simulink model "MotionLab_DigitalTwin"  (R2024b)
settings: Solver=ode3  StartTime=0.0  StopTime=inf  FixedStep=Ts  RelTol=1e-3  AbsTol=1e-3
model workspace: external: MATLAB File .\Parameters.m (data not in the file)
values from neighbouring files (symbols this model uses):
  L2 = 830e-3    (= 0.83)    [Robot_parameters.m]
  L3 = 1160e-3    (= 1.16)    [Robot_parameters.m]
  L4 = 250e-3    (= 0.25)    [Robot_parameters.m]
undefined symbols (not defined in the file or in its folder): smiData, smiDataBig, smiDataBigTop, smiDataRobot, Var, X, Y, Z
libraries: sm_lib x490, nesl_utility x87, slrealtimeutilitieslib x1, slrealtimeiplib x1, aerolibanimutils x1
(part 4 of 15)

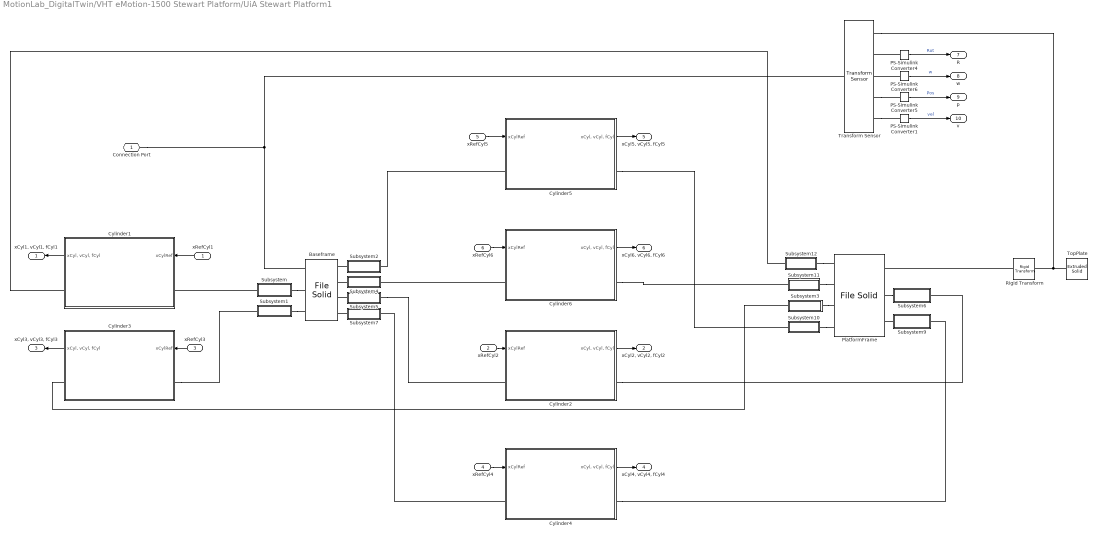
== system MotionLab_DigitalTwin/VHT eMotion-1500 Stewart Platform/UiA Stewart Platform1 ==
  xRefCyl1 : Inport
  xRefCyl2 : Inport  Port=2
  xRefCyl3 : Inport  Port=3
  xRefCyl4 : Inport  Port=4
  xRefCyl5 : Inport  Port=5
  xRefCyl6 : Inport  Port=6
  Baseframe : sm_lib/Body Elements/File Solid  ExtGeomFileName=.\CAD_Lille\1400_Derived Baseframe_crdincl.stp_Default_sldprt.STEP  UnitType=FromFile  ExtGeomFileUnits=m  StepReaderType=HEX  ExportConvexHullGeometry=off  InertiaType=Custom  BasedOnType=DensityFromFile  Density=1000  DensityUnits=kg/m^3  Mass=smiData.Solid(2).mass  MassUnits=kg  CenterOfMass=smiData.Solid(2).CoM  CenterOfMassUnits=mm  MomentsOfInertia=smiData.Solid(2).MoI  MomentsOfInertiaUnits=kg*mm^2  ProductsOfInertia=smiData.Solid(2).PoI  ProductsOfInertiaUnits=kg*mm^2  GraphicType=FromGeometry  MarkerShape=Sphere  MarkerSize=10  GraphicVisPropType=SimpleVisualProperties  GraphicDiffuseColor=[0.2 0.2 0.2]  GraphicOpacity=smiData.Solid(2).opacity  GraphicSpecularColor=[0.5 0.5 0.5 1.0]  GraphicAmbientColor=[0.15 0.15 0.15 1.0]  GraphicEmissiveColor=[0.0 0.0 0.0 1.0]  GraphicShininess=75  DoExposeReferenceFrame=on  SerializedFrames=<Frames><Frame><Id>Frame1</Id><Value><Name>F1</Name><Origin><Source>GeometricFeature</Source><FeatureName>planar surface 569</FeatureName></Origin><PrimaryAxis><DefinedDirection>+Z</DefinedDirection><Source>GeometricFeature</Source><SourceDirection>+Z</SourceDirection><FeatureName>planar surface 569</FeatureName></PrimaryAxis><SecondaryAxis><DefinedDirection>+X</DefinedDirection><Source>ReferenceFrame</Source><SourceDirection>+X</SourceDirection><FeatureName></FeatureName></SecondaryAxis></Value></Frame><Frame><Id>Frame2</Id><Value><Name>F2</Name><Origin><Source>GeometricFeature</Source><FeatureName>planar surface 568</FeatureName></Origin><PrimaryAxis><DefinedDirection>+Z</DefinedDirection><Source>GeometricFeature</Source><SourceDirection>+Z</SourceDirection><FeatureName>planar surface 568</FeatureName></PrimaryAxis><SecondaryAxis><DefinedDirection>+X</DefinedDirection><Source>ReferenceFrame</Source><SourceDirection>+X</SourceDirection><FeatureName></FeatureName></SecondaryAxis></Value></Frame><Frame><Id>Frame3</Id><Value><Name>F3</Name><Origin><Source>GeometricFeature</Source><FeatureName>planar surface 1053</FeatureName></Origin><PrimaryAxis><DefinedDirection>+Z</DefinedDirection><Source>GeometricFeature</Source><SourceDirection>+Z</SourceDirection><FeatureName>planar surface 1053</FeatureName></PrimaryAxis><SecondaryAxis><DefinedDirection>+X</DefinedDirection><Source>ReferenceFrame</Source><SourceDirection>+X</SourceDirection><FeatureName></FeatureName></SecondaryAxis></Value></Frame><Frame><Id>Frame4</Id><Value><Name>F4</Name><Origin><Source>GeometricFeature</Source><FeatureName>planar surface 1052</FeatureName></Origin><PrimaryAxis><DefinedDirection>+Z</DefinedDirection><Source>GeometricFeature</Source><SourceDirection>+Z</SourceDirection><FeatureName>planar surface 1052</FeatureName></PrimaryAxis><SecondaryAxis><DefinedDirection>+X</DefinedDirection><Source>ReferenceFrame</Source><SourceDirection>+X</SourceDirection><FeatureName></FeatureName></SecondaryAxis></Value></Frame><Frame><Id>Frame5</Id><Value><Name>F5</Name><Origin><Source>GeometricFeature</Source><FeatureName>planar surface 907</FeatureName></Origin><PrimaryAxis><DefinedDirection>+Z</DefinedDirection><Source>GeometricFeature</Source><SourceDirection>+Z</SourceDirection><FeatureName>planar surface 907</FeatureName></PrimaryAxis><SecondaryAxis><DefinedDirection>+X</DefinedDirection><Source>ReferenceFrame</Source><SourceDirection>+X</SourceDirection><FeatureName></FeatureName></SecondaryAxis></Value></Frame><Frame><Id>Frame6</Id><Value><Name>F6</Name><Origin><Source>GeometricFeature</Source><FeatureName>planar surface 906</FeatureName></Origin><PrimaryAxis><DefinedDirection>+Z</DefinedDirection><Source>GeometricFeature</Source><SourceDirection>+Z</SourceDirection><FeatureName>planar surface 906</FeatureName></PrimaryAxis><SecondaryAxis><DefinedDirection>+X</DefinedDirection><Source>ReferenceFrame</Source><SourceDirection>+X</SourceDirection><FeatureName></FeatureName></SecondaryAxis></Value></Frame></Frames>
  Cylinder1 : Subsystem
  Cylinder2 : Subsystem
  Cylinder3 : Subsystem
  Cylinder4 : Subsystem
  Cylinder5 : Subsystem
  Cylinder6 : Subsystem
  PS-Simulink Converter{1,4..6} (4 alike) : nesl_utility/PS-Simulink Converter  PhysicalDomain=network_engine_domain  SubClassName=ps_output  LeftPortType=input  RightPortType=output  PseudoPeriodic=off  Frequencies=[]  VectorFormat=inherit  Unit=inherit  AffineConversion=off
  PlatformFrame : sm_lib/Body Elements/File Solid  ExtGeomFileName=.\CAD_Lille\1100_Derived Platfrom_crdincl.stp_Default_sldprt.STEP  UnitType=FromFile  ExtGeomFileUnits=m  StepReaderType=HEX  ExportConvexHullGeometry=off  InertiaType=Custom  BasedOnType=DensityFromFile  Density=1000  DensityUnits=kg/m^3  Mass=smiData.Solid(4).mass  MassUnits=kg  CenterOfMass=smiData.Solid(4).CoM  CenterOfMassUnits=mm  MomentsOfInertia=smiData.Solid(4).MoI  MomentsOfInertiaUnits=kg*mm^2  ProductsOfInertia=smiData.Solid(4).PoI  ProductsOfInertiaUnits=kg*mm^2  GraphicType=FromGeometry  MarkerShape=Sphere  MarkerSize=10  GraphicVisPropType=SimpleVisualProperties  GraphicDiffuseColor=[0.2 0.2 0.2]  GraphicOpacity=1  GraphicSpecularColor=[0.5 0.5 0.5 1.0]  GraphicAmbientColor=[0.15 0.15 0.15 1.0]  GraphicEmissiveColor=[0.0 0.0 0.0 1.0]  GraphicShininess=75  DoExposeReferenceFrame=on  SerializedFrames=<Frames><Frame><Id>Frame1</Id><Value><Name>F1</Name><Origin><Source>GeometricFeature</Source><FeatureName>planar surface 875</FeatureName></Origin><PrimaryAxis><DefinedDirection>+Z</DefinedDirection><Source>GeometricFeature</Source><SourceDirection>+Z</SourceDirection><FeatureName>planar surface 875</FeatureName></PrimaryAxis><SecondaryAxis><DefinedDirection>+X</DefinedDirection><Source>ReferenceFrame</Source><SourceDirection>+X</SourceDirection><FeatureName></FeatureName></SecondaryAxis></Value></Frame><Frame><Id>Frame2</Id><Value><Name>F2</Name><Origin><Source>GeometricFeature</Source><FeatureName>planar surface 858</FeatureName></Origin><PrimaryAxis><DefinedDirection>+Z</DefinedDirection><Source>GeometricFeature</Source><SourceDirection>+Z</SourceDirection><FeatureName>planar surface 858</FeatureName></PrimaryAxis><SecondaryAxis><DefinedDirection>+X</DefinedDirection><Source>ReferenceFrame</Source><SourceDirection>+X</SourceDirection><FeatureName></FeatureName></SecondaryAxis></Value></Frame><Frame><Id>Frame3</Id><Value><Name>F3</Name><Origin><Source>GeometricFeature</Source><FeatureName>planar surface 428</FeatureName></Origin><PrimaryAxis><DefinedDirection>+Z</DefinedDirection><Source>GeometricFeature</Source><SourceDirection>+Z</SourceDirection><FeatureName>planar surface 428</FeatureName></PrimaryAxis><SecondaryAxis><DefinedDirection>+X</DefinedDirection><Source>ReferenceFrame</Source><SourceDirection>+X</SourceDirection><FeatureName></FeatureName></SecondaryAxis></Value></Frame><Frame><Id>Frame4</Id><Value><Name>F4</Name><Origin><Source>GeometricFeature</Source><FeatureName>planar surface 274</FeatureName></Origin><PrimaryAxis><DefinedDirection>+Z</DefinedDirection><Source>GeometricFeature</Source><SourceDirection>+Z</SourceDirection><FeatureName>planar surface 274</FeatureName></PrimaryAxis><SecondaryAxis><DefinedDirection>+X</DefinedDirection><Source>ReferenceFrame</Source><SourceDirection>+X</SourceDirection><FeatureName></FeatureName></SecondaryAxis></Value></Frame><Frame><Id>Frame5</Id><Value><Name>F5</Name><Origin><Source>GeometricFeature</Source><FeatureName>planar surface 892</FeatureName></Origin><PrimaryAxis><DefinedDirection>+Z</DefinedDirection><Source>GeometricFeature</Source><SourceDirection>+Z</SourceDirection><FeatureName>planar surface 892</FeatureName></PrimaryAxis><SecondaryAxis><DefinedDirection>+X</DefinedDirection><Source>ReferenceFrame</Source><SourceDirection>+X</SourceDirection><FeatureName></FeatureName></SecondaryAxis></Value></Frame><Frame><Id>Frame6</Id><Value><Name>F6</Name><Origin><Source>GeometricFeature</Source><FeatureName>planar surface 909</FeatureName></Origin><PrimaryAxis><DefinedDirection>+Z</DefinedDirection><Source>GeometricFeature</Source><SourceDirection>+Z</SourceDirection><FeatureName>planar surface 909</FeatureName></PrimaryAxis><SecondaryAxis><DefinedDirection>+X</DefinedDirection><Source>ReferenceFrame</Source><SourceDirection>+X</SourceDirection><FeatureName></FeatureName></SecondaryAxis></Value></Frame></Frames>
  Rigid Transform : sm_lib/Frames and Transforms/Rigid Transform  RotationMethod=None  FollAlignAxisA=+X  BaseAlignAxisA=+Y  FollAlignAxisB=+Y  BaseAlignAxisB=+Z  RotationStandardAxis=+Z  RotationAngle=0.0  RotationAngleUnits=deg  RotationArbitraryAxis=[0 0 1]  RotationSequenceAxes=FollowerAxes  RotationSequence=XYX  RotationSequenceAngles=[0 0 0]  RotationSequenceAnglesUnits=deg  RotationMatrix=[1 0 0; 0 1 0; 0 0 1]  Quaternion=[1 0 0 0]  TranslationMethod=StandardAxis  TranslationCartesianOffset=[0 0 0]  TranslationCartesianOffsetUnits=m  TranslationStandardAxis=+Z  TranslationStandardOffset=190  TranslationStandardOffsetUnits=mm  TranslationROffset=0  TranslationROffsetUnits=m  TranslationThetaOffset=0  TranslationThetaOffsetUnits=deg  TranslationZOffset=0  TranslationZOffsetUnits=m
  Subsystem : Subsystem
  Subsystem1 : Subsystem
  Subsystem10 : Subsystem
  Subsystem11 : Subsystem
  Subsystem12 : Subsystem
  Subsystem2 : Subsystem
  Subsystem3 : Subsystem
  Subsystem4 : Subsystem
  Subsystem5 : Subsystem
  Subsystem6 : Subsystem
  Subsystem7 : Subsystem
  Subsystem9 : Subsystem
  TopPlate : sm_lib/Body Elements/Extruded Solid  ExtrusionType=Regular  PolygonNumSides=3  PolygonOuterRadius=1.366  PolygonOuterRadiusUnits=m  ExportEntireGeometry=off  ExtrusionCrossSection=[1 1; -1 1; -1 -1; 1 -1]  ExtrusionCrossSectionUnits=m  ExportConvexHullGeometry=off  ExtrusionLength=10  ExtrusionLengthUnits=mm  InertiaType=CalculateFromGeometry  BasedOnType=Density  Density=7800  DensityUnits=kg/m^3  Mass=1  MassUnits=kg  CenterOfMass=[0 0 0]  CenterOfMassUnits=m  MomentsOfInertia=[1 1 1]  MomentsOfInertiaUnits=kg*m^2  ProductsOfInertia=[0 0 0]  ProductsOfInertiaUnits=kg*m^2  GraphicType=FromGeometry  MarkerShape=Sphere  MarkerSize=10  GraphicVisPropType=SimpleVisualProperties  GraphicDiffuseColor=[0.4 0.4 0.4]  GraphicOpacity=1.0  GraphicSpecularColor=[0.5 0.5 0.5 1.0]  GraphicAmbientColor=[0.15 0.15 0.15 1.0]  GraphicEmissiveColor=[0.0 0.0 0.0 1.0]  GraphicShininess=75  DoExposeReferenceFrame=on  SerializedFrames=<Frames/>
  Transform Sensor : sm_lib/Frames and Transforms/Transform Sensor  MeasurementFrame=Base  RotationSequence=ZYX  SenseAngle=off  SenseAxis=off  SenseQ=off  SenseR=on  SenseRotationSequence=off  SenseOmegaX=off  SenseOmegaY=off  SenseOmegaZ=off  SenseOmega=on  SenseQDot=off  SenseRDot=off  SenseRotationSequenceDot=off  SenseAlphaX=off  SenseAlphaY=off  SenseAlphaZ=off  SenseAlpha=off  SenseQDDot=off  SenseRDDot=off  SenseX=off  SenseY=off  SenseZ=off  SenseXYZ=on  SenseRad=off  SenseAzim=off  SenseDist=off  SenseInc=off  SenseXDot=off  SenseYDot=off  SenseZDot=off  SenseXYZDot=on  SenseRadDot=off  SenseAzimDot=off  SenseDistDot=off  SenseIncDot=off  SenseXDDot=off  SenseYDDot=off  SenseZDDot=off  SenseXYZDDot=off  SenseRadDDot=off  SenseAzimDDot=off  SenseDistDDot=off  SenseIncDDot=off
  Connection Port : PMIOPort  Side=Left
  "xCyl1, vCyl1, fCyl1" : Outport
  "xCyl2, vCyl2, fCyl2" : Outport  Port=2
  "xCyl3, vCyl3, fCyl3" : Outport  Port=3
  "xCyl4, vCyl4, fCyl4" : Outport  Port=4
  "xCyl5, vCyl5, fCyl5" : Outport  Port=5
  "xCyl6, vCyl6, fCyl6" : Outport  Port=6
  R : Outport  Port=7
  w : Outport  Port=8
  p : Outport  Port=9
  v : Outport  Port=10
  wires:
  Cylinder5/1("xCyl, vCyl, fCyl") -> "xCyl5, vCyl5, fCyl5"/1
  Cylinder6/1("xCyl, vCyl, fCyl") -> "xCyl6, vCyl6, fCyl6"/1
  Cylinder2/1("xCyl, vCyl, fCyl") -> "xCyl2, vCyl2, fCyl2"/1
  Cylinder4/1("xCyl, vCyl, fCyl") -> "xCyl4, vCyl4, fCyl4"/1
  Cylinder3/1("xCyl, vCyl, fCyl") -> "xCyl3, vCyl3, fCyl3"/1
  Cylinder1/1("xCyl, vCyl, fCyl") -> "xCyl1, vCyl1, fCyl1"/1
  PS-Simulink Converter5/1 -> p/1  "Pos"
  PS-Simulink Converter6/1 -> w/1  "w"
  PS-Simulink Converter4/1 -> R/1  "Rot"
  xRefCyl3/1 -> Cylinder3/1(xCylRef)
  xRefCyl1/1 -> Cylinder1/1(xCylRef)
  xRefCyl2/1 -> Cylinder2/1(xCylRef)
  xRefCyl6/1 -> Cylinder6/1(xCylRef)
  xRefCyl5/1 -> Cylinder5/1(xCylRef)
  xRefCyl4/1 -> Cylinder4/1(xCylRef)
  PS-Simulink Converter1/1 -> v/1  "vel"
  connections:
  Subsystem5/RConn1 -- Cylinder2/LConn1
  PlatformFrame/RConn2 -- Subsystem6/LConn1
  Cylinder6/RConn1 -- Subsystem11/RConn1
  Cylinder5/LConn1 -- Subsystem2/RConn1
  Cylinder4/LConn1 -- Subsystem7/RConn1
  Cylinder3/LConn1 -- Subsystem1/RConn1
  Cylinder2/RConn1 -- Subsystem6/RConn1
  Subsystem12/RConn1 -- Cylinder1/RConn1
  Subsystem3/RConn1 -- Cylinder3/RConn1
  Cylinder6/LConn1 -- Subsystem4/RConn1
  Subsystem9/LConn1 -- PlatformFrame/RConn3
  Subsystem12/LConn1 -- PlatformFrame/LConn1
  Subsystem10/LConn1 -- PlatformFrame/LConn4
  Cylinder4/RConn1 -- Subsystem9/RConn1
  Subsystem3/LConn1 -- PlatformFrame/LConn3
  Subsystem11/LConn1 -- PlatformFrame/LConn2
  Cylinder5/RConn1 -- Subsystem10/RConn1
  Rigid Transform/LConn1 -- PlatformFrame/RConn1
  Transform Sensor/LConn1 -- Baseframe/RConn1 -- Connection Port/RConn1
  PS-Simulink Converter4/LConn1 -- Transform Sensor/RConn2
  Subsystem/LConn1 -- Baseframe/RConn2
  Subsystem/RConn1 -- Cylinder1/LConn1
  Subsystem1/LConn1 -- Baseframe/RConn3
  Subsystem2/LConn1 -- Baseframe/LConn1
  Subsystem4/LConn1 -- Baseframe/LConn2
  Subsystem5/LConn1 -- Baseframe/LConn3
  Subsystem7/LConn1 -- Baseframe/LConn4
  Transform Sensor/RConn4 -- PS-Simulink Converter5/LConn1
  PS-Simulink Converter6/LConn1 -- Transform Sensor/RConn3
  Transform Sensor/RConn5 -- PS-Simulink Converter1/LConn1
  TopPlate/RConn1 -- Transform Sensor/RConn1 -- Rigid Transform/RConn1

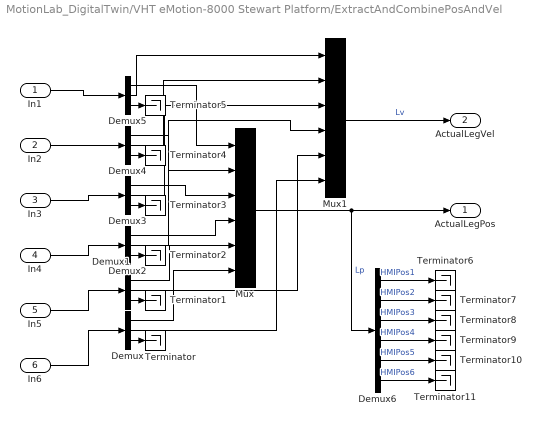
== system MotionLab_DigitalTwin/VHT eMotion-8000 Stewart Platform/ExtractAndCombinePosAndVel ==
  In1 : Inport
  In2 : Inport  Port=2
  In3 : Inport  Port=3
  In4 : Inport  Port=4
  In5 : Inport  Port=5
  In6 : Inport  Port=6
  Demux{,1..5} (6 alike) : Demux  Outputs=3
  Demux6 : Demux  Outputs=6
  Mux : Mux  Inputs=6
  Mux1 : Mux  Inputs=6
  Terminator{,1..11} (12 alike) : Terminator
  ActualLegPos : Outport
  ActualLegVel : Outport  Port=2
  wires:
  Demux1/1 -> Mux/5
  Demux4/1 -> Mux/2
  Demux4/2 -> Mux1/2
  Demux3/1 -> Mux/3
  Demux3/2 -> Mux1/3
  Mux1/1 -> ActualLegVel/1  "Lv"
  Demux5/1 -> Mux/1
  Demux2/1 -> Mux/4
  In4/1 -> Demux2/1
  Demux5/2 -> Mux1/1
  Demux/1 -> Mux/6
  Demux2/2 -> Mux1/4
  Demux/2 -> Mux1/6
  Demux1/2 -> Mux1/5
  In1/1 -> Demux5/1
  In6/1 -> Demux/1
  In3/1 -> Demux3/1
  In5/1 -> Demux1/1
  In2/1 -> Demux4/1
  Mux/1 -> ActualLegPos/1, Demux6/1  "Lp"
  Demux/3 -> Terminator/1
  Demux1/3 -> Terminator1/1
  Demux2/3 -> Terminator2/1
  Demux3/3 -> Terminator3/1
  Demux4/3 -> Terminator4/1
  Demux5/3 -> Terminator5/1
  Demux6/1 -> Terminator6/1  "HMIPos1"
  Demux6/2 -> Terminator7/1  "HMIPos2"
  Demux6/3 -> Terminator8/1  "HMIPos3"
  Demux6/4 -> Terminator9/1  "HMIPos4"
  Demux6/5 -> Terminator10/1  "HMIPos5"
  Demux6/6 -> Terminator11/1  "HMIPos6"

== system MotionLab_DigitalTwin/VHT eMotion-8000 Stewart Platform/Inverse Kinematics ==
  RotBig : Inport
  wBig : Inport  Port=2
  posBig : Inport  Port=3
  velBig : Inport  Port=4
  Demux2 : Demux  Outputs=6
  Gain : Gain  Gain=-1
  InvKin : MATLAB Function  TreatAsAtomicUnit=on
  InvKin1 : MATLAB Function  Commented=on  TreatAsAtomicUnit=on
  y : Outport
  y1 : Outport  Port=2
  xRefCyl1 : Outport  Port=3
  xRefCyl2 : Outport  Port=4
  xRefCyl3 : Outport  Port=5
  xRefCyl4 : Outport  Port=6
  xRefCyl5 : Outport  Port=7
  xRefCyl6 : Outport  Port=8
  wires:
  InvKin/1(f) -> Gain/1  "InvPos"
  InvKin/2(g) -> y1/1  "InvVel"
  RotBig/1 -> InvKin/1(RotBig)  "Top_Rot"
  wBig/1 -> InvKin/2(wBig)  "Top_W"
  posBig/1 -> InvKin/3(posBig)  "Top_Pos"
  velBig/1 -> InvKin/4(velBig)  "Top_Vel"
  Demux2/6 -> xRefCyl6/1
  Demux2/2 -> xRefCyl2/1
  Demux2/1 -> xRefCyl1/1
  Demux2/3 -> xRefCyl3/1
  Demux2/5 -> xRefCyl5/1
  Demux2/4 -> xRefCyl4/1
  Gain/1 -> Demux2/1, y/1

== system MotionLab_DigitalTwin/VHT eMotion-8000 Stewart Platform/MBS Config ==
  Floor : sm_lib/Body Elements/Brick Solid  BrickDimensions=[17 12 0.001]  BrickDimensionsUnits=m  ExportEntireGeometry=off  InertiaType=CalculateFromGeometry  BasedOnType=Density  Density=1000  DensityUnits=kg/m^3  Mass=1  MassUnits=kg  CenterOfMass=[0 0 0]  CenterOfMassUnits=m  MomentsOfInertia=[1 1 1]  MomentsOfInertiaUnits=kg*m^2  ProductsOfInertia=[0 0 0]  ProductsOfInertiaUnits=kg*m^2  GraphicType=FromGeometry  MarkerShape=Sphere  MarkerSize=10  GraphicVisPropType=SimpleVisualProperties  GraphicDiffuseColor=[1.0 1.0 1.0]  GraphicOpacity=1  GraphicSpecularColor=[0.5 0.5 0.5 1.0]  GraphicAmbientColor=[0.15 0.15 0.15 1.0]  GraphicEmissiveColor=[0.0 0.0 0.0 1.0]  GraphicShininess=75  DoExposeReferenceFrame=on  SerializedFrames=<Frames/>
  Mechanism Configuration1 : sm_lib/Utilities/Mechanism Configuration  UniformGravity=Constant  GravityVector=[0 0 -9.80665]  GravityVectorUnits=m/s^2  LinearizationDelta=0.001  JointModeTransitionNonlinearIterations=2
  Solver Configuration1 : nesl_utility/Solver Configuration  PhysicalDomain=network_engine_domain  SubClassName=solver  LeftPortType=input  RightPortType=generic  Tones=[]  Harmonics=[]  SimulateNoise=off  Profile=off  UseLocalSampling=off  EnableSwitchedLinearOptims=on  FrequencyDomain=off  UseCCode=off  RelTol=0.001  AbsTol=1e-06  MinStep=1e-09  ToWorkspace=off  RevertToSquareIcSolve=off  NumHomotopyIterations=100  PhasorMode=off  PhasorModeNumHarmonics=1  ConsistencySolver=NEWTON_XTOL_AFTER_FTOL  IndexReductionMethod=DerivativeReplacement  DoDC=off  ResidualTolerance=1e-09  ConsistencyTolSource=GLOBAL  ConsistencyAbsTol=0.001  ConsistencyRelTol=0.001  ConsistencyTolFactor=0.02  UseLocalSolver=off  LocalSolverChoice=NE_BACKWARD_EULER_ADVANCER  ResolveIndetEquations=on  FunctionEvalNumThread=1  LocalSolverSampleTime=0.001  DoFixedCost=off  MaxNonlinIter=3  MaxModeIter=2  ComputeImpulses=off  ImpulseIterations=2  LinearAlgebra=auto  LinearAlgebraNumThread=0  EquationFormulation=NE_TIME_EF  DelaysMemoryBudget=1024  AutomaticFiltering=on  FilteringTimeConstant=0.001  PartitionStorageMethod=AS_NEEDED  PartitionMemoryBudget=1024  PartitionMethod=ROBUST  MultibodyUseLocalSolver=off  MultibodyLocalSolverChoice=ODE2  MultibodyLocalSolverSampleTime=0.02
  World Frame1 : sm_lib/Frames and Transforms/World Frame
  Out : PMIOPort  Side=Right
  connections:
  Solver Configuration1/RConn1 -- Floor/RConn1 -- Out/RConn1 -- Mechanism Configuration1/RConn1 -- World Frame1/RConn1

== system MotionLab_DigitalTwin/VHT eMotion-8000 Stewart Platform/Motion Control System ==
  em8000_UDP : Inport
  Constant : Constant  Value=0.751
  Demux : Demux  Outputs=6
  MotionGen : MATLAB Function  TreatAsAtomicUnit=on
  Sum : Sum  Inputs=|++
  Velocity Calculation : Subsystem
  R_top : Outport
  w_top : Outport  Port=2
  ptop : Outport  Port=3
  v_top : Outport  Port=4
  wires:
  MotionGen/3(p_top) -> ptop/1  "ptop"
  MotionGen/2(R_top) -> R_top/1  "R_top"
  MotionGen/1(motion) -> Velocity Calculation/1(generated motion)  "generated motion"
  Velocity Calculation/1(w_top) -> w_top/1
  Velocity Calculation/2(v_top) -> v_top/1
  Demux/1 -> MotionGen/1(surge)
  Demux/2 -> MotionGen/2(sway)
  Demux/4 -> MotionGen/4(roll)
  Demux/5 -> MotionGen/5(pitch)
  Demux/6 -> MotionGen/6(yaw)
  em8000_UDP/1 -> Demux/1
  Demux/3 -> Sum/1
  Sum/1 -> MotionGen/3(heave)
  Constant/1 -> Sum/2

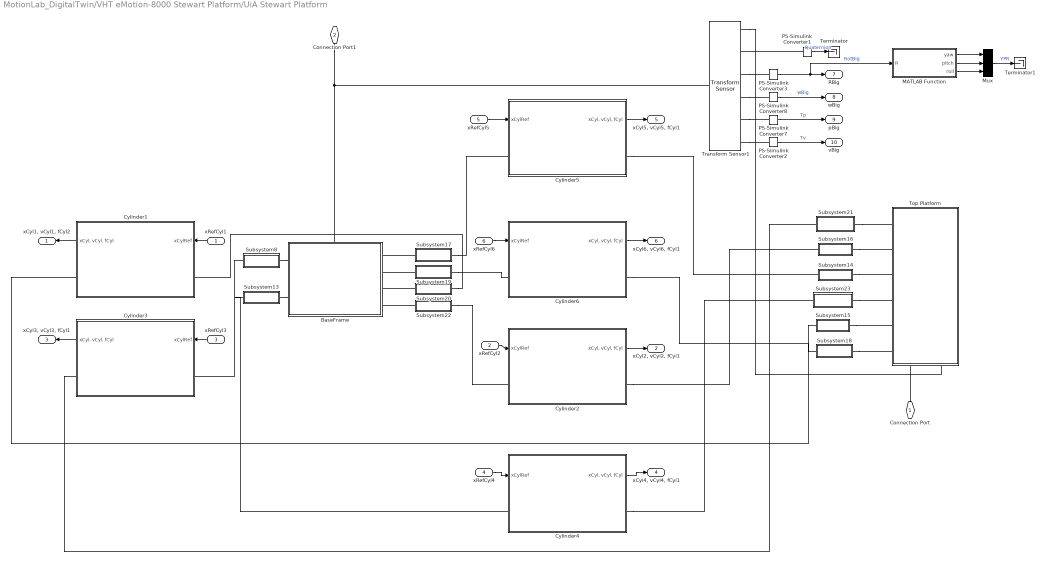
== system MotionLab_DigitalTwin/VHT eMotion-8000 Stewart Platform/UiA Stewart Platform ==
  xRefCyl1 : Inport
  xRefCyl2 : Inport  Port=2
  xRefCyl3 : Inport  Port=3
  xRefCyl4 : Inport  Port=4
  xRefCyl5 : Inport  Port=5
  xRefCyl6 : Inport  Port=6
  BaseFrame : Subsystem
      settings: PortSchema="{\"entries\":[{\"content\":{\"sides\":[{\"content\":{\"connectorIds\":[\"LConn1\",\"LConn2\"]},\"type\":\"ConnectorPlacement.EquallySpacedRectSide\",\"uuid\":\"da4ab1d9-b03b-4752-96dc-d461d460a286\"},{\"content\":{\"connectorIds\":[\"RConn1\",\"RConn2\",\"RConn3\",\"RConn4\"],\"side\":\"RIGHT\"},\"type\":\"ConnectorPlacement.EquallySpacedRectSide\",\"uuid\":\"73e2cee5-e579-4799-a91d-51d3e83bff98\"},{\"content\":{\"connectorIds\":[\"LConn3\"],\"side\":\"TOP\"},\"type\":\"ConnectorPlacement.EquallySpacedRectSide\",\"uuid\":\"06df1dd1-a0d0-4e1d-989b-9b685334890f\"}]},\"type\":\"ConnectorPlacement.EquallySpacedConnector\",\"uuid\":\"bc5837cf-a25b-4221-8240-81057aa0f393\"}],\"packageUris\":[\"http://schema.mathworks.com/mf0/Connector/R2020b\"],\"version\":\"1.0\"}"
  Cylinder1 : Subsystem
  Cylinder2 : Subsystem
  Cylinder3 : Subsystem
  Cylinder4 : Subsystem
  Cylinder5 : Subsystem
  Cylinder6 : Subsystem
  MATLAB Function : MATLAB Function  TreatAsAtomicUnit=on
  Mux : Mux  Inputs=3
  PS-Simulink Converter{1..3,7..8} (5 alike) : nesl_utility/PS-Simulink Converter  PhysicalDomain=network_engine_domain  SubClassName=ps_output  LeftPortType=input  RightPortType=output  PseudoPeriodic=off  Frequencies=[]  VectorFormat=inherit  Unit=inherit  AffineConversion=off
  Subsystem13 : Subsystem
  Subsystem14 : Subsystem
  Subsystem15 : Subsystem
  Subsystem16 : Subsystem
  Subsystem17 : Subsystem
  Subsystem18 : Subsystem
  Subsystem19 : Subsystem
  Subsystem20 : Subsystem
  Subsystem21 : Subsystem
  Subsystem22 : Subsystem
  Subsystem23 : Subsystem
  Subsystem8 : Subsystem
  Terminator : Terminator
  Terminator1 : Terminator
  Top Platform : Subsystem
      settings: PortSchema="{\"entries\":[{\"content\":{\"sides\":[{\"content\":{},\"type\":\"ConnectorPlacement.EquallySpacedRectSide\",\"uuid\":\"ca3217db-4e20-489f-a6cd-b1724b78efd3\"},{\"content\":{\"connectorIds\":[\"RConn1\",\"RConn2\",\"RConn3\",\"RConn4\",\"RConn5\",\"RConn6\"],\"side\":\"RIGHT\"},\"type\":\"ConnectorPlacement.EquallySpacedRectSide\",\"uuid\":\"fd1e2a43-5c5d-4894-9378-ab9ed15d0301\"},{\"content\":{\"connectorIds\":[\"LConn1\",\"LConn2\"],\"side\":\"TOP\"},\"type\":\"ConnectorPlacement.EquallySpacedRectSide\",\"uuid\":\"5dcdcf64-3199-48e6-a5b7-dbaa81855341\"}]},\"type\":\"ConnectorPlacement.EquallySpacedConnector\",\"uuid\":\"ca4b8478-096a-42c6-929b-3f00269cdec9\"}],\"packageUris\":[\"http://schema.mathworks.com/mf0/Connector/R2020b\"],\"version\":\"1.0\"}"
  Transform Sensor1 : sm_lib/Frames and Transforms/Transform Sensor  MeasurementFrame=Base  RotationSequence=ZYX  SenseAngle=off  SenseAxis=off  SenseQ=on  SenseR=on  SenseRotationSequence=off  SenseOmegaX=off  SenseOmegaY=off  SenseOmegaZ=off  SenseOmega=on  SenseQDot=off  SenseRDot=off  SenseRotationSequenceDot=off  SenseAlphaX=off  SenseAlphaY=off  SenseAlphaZ=off  SenseAlpha=off  SenseQDDot=off  SenseRDDot=off  SenseX=off  SenseY=off  SenseZ=off  SenseXYZ=on  SenseRad=off  SenseAzim=off  SenseDist=off  SenseInc=off  SenseXDot=off  SenseYDot=off  SenseZDot=off  SenseXYZDot=on  SenseRadDot=off  SenseAzimDot=off  SenseDistDot=off  SenseIncDot=off  SenseXDDot=off  SenseYDDot=off  SenseZDDot=off  SenseXYZDDot=off  SenseRadDDot=off  SenseAzimDDot=off  SenseDistDDot=off  SenseIncDDot=off
  Connection Port : PMIOPort  Side=Left
  Connection Port1 : PMIOPort  Port=2  Side=Left
  "xCyl1, vCyl1, fCyl2" : Outport
  "xCyl2, vCyl2, fCyl1" : Outport  Port=2
  "xCyl3, vCyl3, fCyl1" : Outport  Port=3
  "xCyl4, vCyl4, fCyl1" : Outport  Port=4
  "xCyl5, vCyl5, fCyl1" : Outport  Port=5
  "xCyl6, vCyl6, fCyl1" : Outport  Port=6
  RBig : Outport  Port=7
  wBig : Outport  Port=8
  pBig : Outport  Port=9
  vBig : Outport  Port=10
  wires:
  PS-Simulink Converter2/1 -> vBig/1  "Tv"
  xRefCyl2/1 -> Cylinder2/1(xCylRef)
  PS-Simulink Converter8/1 -> wBig/1  "wBig"
  xRefCyl1/1 -> Cylinder1/1(xCylRef)
  Cylinder3/1("xCyl, vCyl, fCyl") -> "xCyl3, vCyl3, fCyl1"/1
  xRefCyl4/1 -> Cylinder4/1(xCylRef)
  PS-Simulink Converter3/1 -> RBig/1, MATLAB Function/1(R)  "RotBig"
  PS-Simulink Converter7/1 -> pBig/1  "Tp"
  Cylinder4/1("xCyl, vCyl, fCyl") -> "xCyl4, vCyl4, fCyl1"/1
  xRefCyl5/1 -> Cylinder5/1(xCylRef)
  Cylinder6/1("xCyl, vCyl, fCyl") -> "xCyl6, vCyl6, fCyl1"/1
  xRefCyl3/1 -> Cylinder3/1(xCylRef)
  Cylinder5/1("xCyl, vCyl, fCyl") -> "xCyl5, vCyl5, fCyl1"/1
  xRefCyl6/1 -> Cylinder6/1(xCylRef)
  Cylinder1/1("xCyl, vCyl, fCyl") -> "xCyl1, vCyl1, fCyl2"/1
  Cylinder2/1("xCyl, vCyl, fCyl") -> "xCyl2, vCyl2, fCyl1"/1
  PS-Simulink Converter1/1 -> Terminator/1  "Quaternion"
  MATLAB Function/1(yaw) -> Mux/1
  MATLAB Function/2(pitch) -> Mux/2
  MATLAB Function/3(roll) -> Mux/3
  Mux/1 -> Terminator1/1  "YPR"
  connections:
  Subsystem20/LConn1 -- BaseFrame/RConn3
  Subsystem13/LConn1 -- BaseFrame/LConn2
  Subsystem22/LConn1 -- BaseFrame/RConn4
  Subsystem17/LConn1 -- BaseFrame/RConn1
  Subsystem19/LConn1 -- BaseFrame/RConn2
  Subsystem8/LConn1 -- BaseFrame/LConn1
  Connection Port1/RConn1 -- BaseFrame/LConn3 -- Transform Sensor1/LConn1
  Subsystem17/RConn1 -- Cylinder5/LConn1
  Subsystem19/RConn1 -- Cylinder6/LConn1
  Subsystem20/RConn1 -- Cylinder1/LConn1
  Subsystem22/RConn1 -- Cylinder2/LConn1
  Subsystem8/RConn1 -- Cylinder3/LConn1
  Subsystem13/RConn1 -- Cylinder4/LConn1
  Transform Sensor1/RConn1 -- Top Platform/LConn1
  Subsystem14/LConn1 -- Top Platform/RConn4
  Subsystem16/LConn1 -- Top Platform/RConn5
  Subsystem21/LConn1 -- Top Platform/RConn6
  Subsystem23/LConn1 -- Top Platform/RConn3
  Subsystem15/LConn1 -- Top Platform/RConn2
  Subsystem18/LConn1 -- Top Platform/RConn1
  Cylinder1/RConn1 -- Subsystem15/RConn1
  Cylinder3/RConn1 -- Subsystem21/RConn1
  Cylinder5/RConn1 -- Subsystem14/RConn1
  Cylinder6/RConn1 -- Subsystem18/RConn1
  Cylinder2/RConn1 -- Subsystem16/RConn1
  Cylinder4/RConn1 -- Subsystem23/RConn1
  Transform Sensor1/RConn3 -- PS-Simulink Converter3/LConn1
  Transform Sensor1/RConn4 -- PS-Simulink Converter8/LConn1
  Transform Sensor1/RConn5 -- PS-Simulink Converter7/LConn1
  Transform Sensor1/RConn6 -- PS-Simulink Converter2/LConn1
  PS-Simulink Converter1/LConn1 -- Transform Sensor1/RConn2
  Connection Port/RConn1 -- Top Platform/LConn2

== system MotionLab_DigitalTwin/ Comau Smart-5 NJ 110-3.0 Industrial Robot/Robot Model/MotorBehind ==
  MotorTop : sm_lib/Body Elements/File Solid  ExtGeomFileName=./CAD_Robot/SMART-5 NJ-110-3.0_CR82350050_SM.STEP_Default_sldprt.STEP  UnitType=FromFile  ExtGeomFileUnits=m  StepReaderType=HEX  ExportConvexHullGeometry=off  InertiaType=Custom  BasedOnType=DensityFromFile  Density=1000  DensityUnits=kg/m^3  Mass=smiDataRobot.Solid(7).mass  MassUnits=kg  CenterOfMass=smiDataRobot.Solid(7).CoM  CenterOfMassUnits=mm  MomentsOfInertia=smiDataRobot.Solid(7).MoI  MomentsOfInertiaUnits=kg*mm^2  ProductsOfInertia=smiDataRobot.Solid(7).PoI  ProductsOfInertiaUnits=kg*mm^2  GraphicType=FromGeometry  MarkerShape=Sphere  MarkerSize=10  GraphicVisPropType=SimpleVisualProperties  GraphicDiffuseColor=[0.2 0.2 0.2]  GraphicOpacity=smiDataRobot.Solid(7).opacity  GraphicSpecularColor=[0.5 0.5 0.5 1.0]  GraphicAmbientColor=[0.15 0.15 0.15 1.0]  GraphicEmissiveColor=[0.0 0.0 0.0 1.0]  GraphicShininess=75  DoExposeReferenceFrame=on  SerializedFrames=<Frames/>
  Rigid Transform7 : sm_lib/Frames and Transforms/Rigid Transform  RotationMethod=StandardAxis  FollAlignAxisA=+X  BaseAlignAxisA=+Y  FollAlignAxisB=+Y  BaseAlignAxisB=+Z  RotationStandardAxis=-Y  RotationAngle=90  RotationAngleUnits=deg  RotationArbitraryAxis=[0 0 1]  RotationSequenceAxes=FollowerAxes  RotationSequence=XYX  RotationSequenceAngles=[0 0 0]  RotationSequenceAnglesUnits=deg  RotationMatrix=[1 0 0; 0 1 0; 0 0 1]  Quaternion=[1 0 0 0]  TranslationMethod=None  TranslationCartesianOffset=[0 0 0]  TranslationCartesianOffsetUnits=m  TranslationStandardAxis=+Z  TranslationStandardOffset=0  TranslationStandardOffsetUnits=m  TranslationROffset=0  TranslationROffsetUnits=m  TranslationThetaOffset=0  TranslationThetaOffsetUnits=deg  TranslationZOffset=0  TranslationZOffsetUnits=m
  Rigid Transform8 : sm_lib/Frames and Transforms/Rigid Transform  RotationMethod=StandardAxis  FollAlignAxisA=+X  BaseAlignAxisA=+Y  FollAlignAxisB=+Y  BaseAlignAxisB=+Z  RotationStandardAxis=-Z  RotationAngle=90  RotationAngleUnits=deg  RotationArbitraryAxis=[0 0 1]  RotationSequenceAxes=FollowerAxes  RotationSequence=XYX  RotationSequenceAngles=[0 0 0]  RotationSequenceAnglesUnits=deg  RotationMatrix=[1 0 0; 0 1 0; 0 0 1]  Quaternion=[1 0 0 0]  TranslationMethod=None  TranslationCartesianOffset=[0 0 0]  TranslationCartesianOffsetUnits=m  TranslationStandardAxis=+Z  TranslationStandardOffset=0  TranslationStandardOffsetUnits=m  TranslationROffset=0  TranslationROffsetUnits=m  TranslationThetaOffset=0  TranslationThetaOffsetUnits=deg  TranslationZOffset=0  TranslationZOffsetUnits=m
  Conn1 : PMIOPort  Side=Left
  connections:
  Rigid Transform7/RConn1 -- Rigid Transform8/LConn1
  Rigid Transform8/RConn1 -- MotorTop/RConn1
  Conn1/RConn1 -- Rigid Transform7/LConn1

== system MotionLab_DigitalTwin/ Comau Smart-5 NJ 110-3.0 Industrial Robot/Robot Model/Motors ==
  MotorLeft : sm_lib/Body Elements/File Solid  ExtGeomFileName=./CAD_Robot/SMART-5 NJ-110-3.0_CR82350070_SM.STEP_Default_sldprt.STEP  UnitType=FromFile  ExtGeomFileUnits=m  StepReaderType=HEX  ExportConvexHullGeometry=off  InertiaType=Custom  BasedOnType=DensityFromFile  Density=1000  DensityUnits=kg/m^3  Mass=smiDataRobot.Solid(9).mass  MassUnits=kg  CenterOfMass=smiDataRobot.Solid(9).CoM  CenterOfMassUnits=mm  MomentsOfInertia=smiDataRobot.Solid(9).MoI  MomentsOfInertiaUnits=kg*mm^2  ProductsOfInertia=smiDataRobot.Solid(9).PoI  ProductsOfInertiaUnits=kg*mm^2  GraphicType=FromGeometry  MarkerShape=Sphere  MarkerSize=10  GraphicVisPropType=SimpleVisualProperties  GraphicDiffuseColor=[0.2 0.2 0.2]  GraphicOpacity=smiDataRobot.Solid(9).opacity  GraphicSpecularColor=[0.5 0.5 0.5 1.0]  GraphicAmbientColor=[0.15 0.15 0.15 1.0]  GraphicEmissiveColor=[0.0 0.0 0.0 1.0]  GraphicShininess=75  DoExposeReferenceFrame=on  SerializedFrames=<Frames/>
  MotorOnTheBack : sm_lib/Body Elements/File Solid  ExtGeomFileName=./CAD_Robot/SMART-5 NJ-110-3.0_CR82350070_SM.STEP_Default_sldprt.STEP  UnitType=FromFile  ExtGeomFileUnits=m  StepReaderType=HEX  ExportConvexHullGeometry=off  InertiaType=Custom  BasedOnType=DensityFromFile  Density=1000  DensityUnits=kg/m^3  Mass=smiDataRobot.Solid(9).mass  MassUnits=kg  CenterOfMass=smiDataRobot.Solid(9).CoM  CenterOfMassUnits=mm  MomentsOfInertia=smiDataRobot.Solid(9).MoI  MomentsOfInertiaUnits=kg*mm^2  ProductsOfInertia=smiDataRobot.Solid(9).PoI  ProductsOfInertiaUnits=kg*mm^2  GraphicType=FromGeometry  MarkerShape=Sphere  MarkerSize=10  GraphicVisPropType=SimpleVisualProperties  GraphicDiffuseColor=[0.2 0.2 0.2]  GraphicOpacity=smiDataRobot.Solid(9).opacity  GraphicSpecularColor=[0.5 0.5 0.5 1.0]  GraphicAmbientColor=[0.15 0.15 0.15 1.0]  GraphicEmissiveColor=[0.0 0.0 0.0 1.0]  GraphicShininess=75  DoExposeReferenceFrame=on  SerializedFrames=<Frames/>
  MotorRight : sm_lib/Body Elements/File Solid  ExtGeomFileName=./CAD_Robot/SMART-5 NJ-110-3.0_CR82350070_SM.STEP_Default_sldprt.STEP  UnitType=FromFile  ExtGeomFileUnits=m  StepReaderType=HEX  ExportConvexHullGeometry=off  InertiaType=Custom  BasedOnType=DensityFromFile  Density=1000  DensityUnits=kg/m^3  Mass=smiDataRobot.Solid(9).mass  MassUnits=kg  CenterOfMass=smiDataRobot.Solid(9).CoM  CenterOfMassUnits=mm  MomentsOfInertia=smiDataRobot.Solid(9).MoI  MomentsOfInertiaUnits=kg*mm^2  ProductsOfInertia=smiDataRobot.Solid(9).PoI  ProductsOfInertiaUnits=kg*mm^2  GraphicType=FromGeometry  MarkerShape=Sphere  MarkerSize=10  GraphicVisPropType=SimpleVisualProperties  GraphicDiffuseColor=[0.2 0.2 0.2]  GraphicOpacity=smiDataRobot.Solid(9).opacity  GraphicSpecularColor=[0.5 0.5 0.5 1.0]  GraphicAmbientColor=[0.15 0.15 0.15 1.0]  GraphicEmissiveColor=[0.0 0.0 0.0 1.0]  GraphicShininess=75  DoExposeReferenceFrame=on  SerializedFrames=<Frames/>
  Rigid Transform1 : sm_lib/Frames and Transforms/Rigid Transform  RotationMethod=StandardAxis  FollAlignAxisA=+X  BaseAlignAxisA=+Y  FollAlignAxisB=+Y  BaseAlignAxisB=+Z  RotationStandardAxis=+X  RotationAngle=180  RotationAngleUnits=deg  RotationArbitraryAxis=[0 0 1]  RotationSequenceAxes=FollowerAxes  RotationSequence=XYX  RotationSequenceAngles=[0 0 0]  RotationSequenceAnglesUnits=deg  RotationMatrix=[1 0 0; 0 1 0; 0 0 1]  Quaternion=[1 0 0 0]  TranslationMethod=StandardAxis  TranslationCartesianOffset=[0 0 0]  TranslationCartesianOffsetUnits=m  TranslationStandardAxis=+Z  TranslationStandardOffset=30  TranslationStandardOffsetUnits=mm  TranslationROffset=0  TranslationROffsetUnits=m  TranslationThetaOffset=0  TranslationThetaOffsetUnits=deg  TranslationZOffset=0  TranslationZOffsetUnits=m
  Rigid Transform2 : sm_lib/Frames and Transforms/Rigid Transform  RotationMethod=StandardAxis  FollAlignAxisA=+X  BaseAlignAxisA=+Y  FollAlignAxisB=+Y  BaseAlignAxisB=+Z  RotationStandardAxis=+X  RotationAngle=180  RotationAngleUnits=deg  RotationArbitraryAxis=[1 0 0]  RotationSequenceAxes=FollowerAxes  RotationSequence=XYX  RotationSequenceAngles=[0 0 0]  RotationSequenceAnglesUnits=deg  RotationMatrix=[1 0 0; 0 1 0; 0 0 1]  Quaternion=[1 0 0 0]  TranslationMethod=StandardAxis  TranslationCartesianOffset=[0 0 0]  TranslationCartesianOffsetUnits=m  TranslationStandardAxis=+Z  TranslationStandardOffset=30  TranslationStandardOffsetUnits=mm  TranslationROffset=0  TranslationROffsetUnits=m  TranslationThetaOffset=0  TranslationThetaOffsetUnits=deg  TranslationZOffset=0  TranslationZOffsetUnits=m
  Rigid Transform3 : sm_lib/Frames and Transforms/Rigid Transform  RotationMethod=StandardAxis  FollAlignAxisA=+X  BaseAlignAxisA=+Y  FollAlignAxisB=+Y  BaseAlignAxisB=+Z  RotationStandardAxis=+Z  RotationAngle=180  RotationAngleUnits=deg  RotationArbitraryAxis=[1 0 0]  RotationSequenceAxes=FollowerAxes  RotationSequence=XYX  RotationSequenceAngles=[0 0 0]  RotationSequenceAnglesUnits=deg  RotationMatrix=[1 0 0; 0 1 0; 0 0 1]  Quaternion=[1 0 0 0]  TranslationMethod=None  TranslationCartesianOffset=[0 0 0]  TranslationCartesianOffsetUnits=m  TranslationStandardAxis=+Z  TranslationStandardOffset=30  TranslationStandardOffsetUnits=mm  TranslationROffset=0  TranslationROffsetUnits=m  TranslationThetaOffset=0  TranslationThetaOffsetUnits=deg  TranslationZOffset=0  TranslationZOffsetUnits=m
  Rigid Transform5 : sm_lib/Frames and Transforms/Rigid Transform  RotationMethod=StandardAxis  FollAlignAxisA=+X  BaseAlignAxisA=+Y  FollAlignAxisB=+Y  BaseAlignAxisB=+Z  RotationStandardAxis=+X  RotationAngle=90  RotationAngleUnits=deg  RotationArbitraryAxis=[0 0 1]  RotationSequenceAxes=FollowerAxes  RotationSequence=XYX  RotationSequenceAngles=[0 0 0]  RotationSequenceAnglesUnits=deg  RotationMatrix=[1 0 0; 0 1 0; 0 0 1]  Quaternion=[1 0 0 0]  TranslationMethod=StandardAxis  TranslationCartesianOffset=[0 0 0]  TranslationCartesianOffsetUnits=m  TranslationStandardAxis=+Y  TranslationStandardOffset=22  TranslationStandardOffsetUnits=mm  TranslationROffset=0  TranslationROffsetUnits=m  TranslationThetaOffset=0  TranslationThetaOffsetUnits=deg  TranslationZOffset=0  TranslationZOffsetUnits=m
  Rigid Transform6 : sm_lib/Frames and Transforms/Rigid Transform  RotationMethod=StandardAxis  FollAlignAxisA=+X  BaseAlignAxisA=+Y  FollAlignAxisB=+Y  BaseAlignAxisB=+Z  RotationStandardAxis=+Z  RotationAngle=30  RotationAngleUnits=deg  RotationArbitraryAxis=[0 0 1]  RotationSequenceAxes=FollowerAxes  RotationSequence=XYX  RotationSequenceAngles=[0 0 0]  RotationSequenceAnglesUnits=deg  RotationMatrix=[1 0 0; 0 1 0; 0 0 1]  Quaternion=[1 0 0 0]  TranslationMethod=None  TranslationCartesianOffset=[0 0 0]  TranslationCartesianOffsetUnits=m  TranslationStandardAxis=+Y  TranslationStandardOffset=22  TranslationStandardOffsetUnits=mm  TranslationROffset=0  TranslationROffsetUnits=m  TranslationThetaOffset=0  TranslationThetaOffsetUnits=deg  TranslationZOffset=0  TranslationZOffsetUnits=m
  Conn1 : PMIOPort  Side=Left
  Conn2 : PMIOPort  Port=2  Side=Left
  Conn3 : PMIOPort  Port=3  Side=Left
  connections:
  Rigid Transform2/LConn1 -- Conn1/RConn1
  Rigid Transform6/LConn1 -- Rigid Transform5/RConn1
  MotorLeft/RConn1 -- Rigid Transform1/RConn1
  MotorRight/RConn1 -- Rigid Transform3/RConn1
  Rigid Transform3/LConn1 -- Rigid Transform2/RConn1
  MotorOnTheBack/RConn1 -- Rigid Transform6/RConn1
  Rigid Transform1/LConn1 -- Conn3/RConn1
  Rigid Transform5/LConn1 -- Conn2/RConn1
